simulink model "anti_windup_DC_motor_R2018a"  (R2018a)
settings: Solver=VariableStepAuto  StartTime=0.0  StopTime=200  RelTol=1e-3
libraries: simulink x1
settings Model: Creator=kjartan  LastModifiedBy=kjartan
settings DataIOCC: ReturnWorkspaceOutputs=on
settings DebuggingCC: SFMachineParentedDataDiag=error
settings SFSimCC: SimUseLocalCustomCode=on
settings RTWCC: RTWUseLocalCustomCode=on

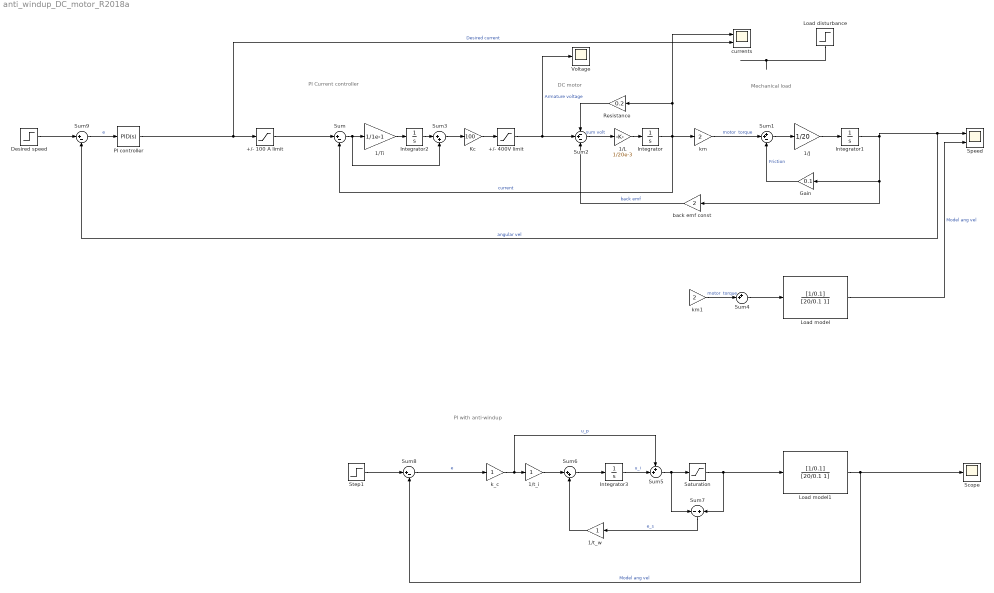
== system anti_windup_DC_motor_R2018a ==
  note: PI with anti-windup
  note: PI Current controller
  note: Mechanical load
  note: DC motor
  +/- 100 A limit : Saturate  UpperLimit=100  LowerLimit=-100
  +/- 400V limit : Saturate  UpperLimit=400  LowerLimit=-400
  1/J : Gain  Gain=1/20
  1/L : Gain  Gain=1/20e-3
  1/Ti : Gain  Gain=1/1e-1
  1/t_i : Gain
  1/t_w : Gain
  Desired speed : Step  Time=0  After=100  SampleTime=0
  Gain : Gain  Gain=0.1
  Integrator{,1..3} (4 alike) : Integrator
  Kc : Gain  Gain=100
  Load disturbance : Step  Time=10  After=10  SampleTime=0
  Load model : TransferFcn  Numerator=[1/0.1]  Denominator=[20/0.1 1]
  Load model1 : TransferFcn  Numerator=[1/0.1]  Denominator=[20/0.1 1]
  PI controller : simulink/Continuous/PID Controller  Controller=PID  Form=Ideal  TimeDomain=Continuous-time  SampleTime=-1  IntegratorMethod=Forward Euler  FilterMethod=Forward Euler  ControllerParametersSource=internal  P=10  I=1/20  D=20  UseFilter=on  N=100  TunerSelectOption=Transfer Function Based (PID Tuner App)  InitialConditionSource=internal  InitialConditionForIntegrator=0  InitialConditionForFilter=0  DifferentiatorICPrevScaledInput=0  ExternalReset=none  TrackingMode=off  Kt=1  LimitOutput=off  UpperSaturationLimit=inf  LowerSaturationLimit=-inf  LinearizeAsGain=on  AntiWindupMode=none  Kb=1  POutMin=[]  POutMax=[]  IOutMin=[]  IOutMax=[]  DOutMin=[]  DOutMax=[]  NOutMin=[]  NOutMax=[]  SumOutMin=[]  SumOutMax=[]  SaturationOutMin=[]  SaturationOutMax=[]  PParamMin=[]  PParamMax=[]  IParamMin=[]  IParamMax=[]  DParamMin=[]  DParamMax=[]  NParamMin=[]  NParamMax=[]  KbParamMin=[]  KbParamMax=[]  KtParamMin=[]  KtParamMax=[]  KbOutMin=[]  KbOutMax=[]  KtOutMin=[]  KtOutMax=[]  IntegratorOutMin=[]  IntegratorOutMax=[]  FilterOutMin=[]  FilterOutMax=[]  SumI1OutMin=[]  SumI1OutMax=[]  SumI2OutMin=[]  SumI2OutMax=[]  SumI3OutMin=[]  SumI3OutMax=[]  SumDOutMin=[]  SumDOutMax=[]  DifferentiatorOutMin=[]  DifferentiatorOutMax=[]  FilterDiffOutCoefMin=[]  FilterDiffOutCoefMax=[]  ReciprocalOutMin=[]  ReciprocalOutMax=[]  SumDenOutMin=[]  SumDenOutMax=[]  SumNumOutMin=[]  SumNumOutMax=[]  DivideOutMin=[]  DivideOutMax=[]  IntegratorContinuousStateAttributes=''  IntegratorStateMustResolveToSignalObject=off  IntegratorRTWStateStorageClass=Auto  FilterContinuousStateAttributes=''  FilterStateMustResolveToSignalObject=off  FilterRTWStateStorageClass=Auto
  Resistance : Gain  Gain=0.2
  Saturation : Saturate
  Scope : Scope
  Speed : Scope  NumInputPorts=2
  Step1 : Step  After=100  SampleTime=0
  Sum : Sum  Inputs=|+-
  Sum1 : Sum  Inputs=++-
  Sum2 : Sum  Inputs=-+-
  Sum3 : Sum  Inputs=|++
  Sum4 : Sum  Inputs=++|
  Sum5 : Sum  Inputs=++|
  Sum6 : Sum  Inputs=|++
  Sum7 : Sum  Inputs=-|+
  Sum8 : Sum  Inputs=|+-
  Sum9 : Sum  Inputs=|+-
  Voltage : Scope
  back emf const : Gain  Gain=2
  currents : Scope  NumInputPorts=2
  k_c : Gain
  km : Gain  Gain=2
  km1 : Gain  Gain=2
  wires:
  Integrator1/1 -> back emf const/1, Gain/1, Sum9/2, Speed/1  "angular vel"
  1/L/1 -> Integrator/1
  Integrator/1 -> Sum/2, currents/1, Resistance/1, km/1  "current"
  km/1 -> Sum1/2  "motor  torque"
  Sum1/1 -> 1/J/1
  1/J/1 -> Integrator1/1
  Gain/1 -> Sum1/3  "Friction"
  Sum2/1 -> 1/L/1  "sum volt"
  back emf const/1 -> Sum2/3  "back emf"
  +/- 400V limit/1 -> Voltage/1, Sum2/2  "Armature voltage"
  Resistance/1 -> Sum2/1
  Kc/1 -> +/- 400V limit/1
  Sum3/1 -> Kc/1
  Integrator2/1 -> Sum3/1
  1/Ti/1 -> Integrator2/1
  Sum/1 -> Sum3/2, 1/Ti/1
  +/- 100 A limit/1 -> Sum/1
  PI controller/1 -> currents/2, +/- 100 A limit/1  "Desired current"
  Load disturbance/1 -> ?
  Sum4/1 -> Load model/1
  Load model/1 -> Speed/2  "Model ang vel"
  Sum5/1 -> Sum7/1, Saturation/1
  Saturation/1 -> Sum7/2, Load model1/1
  Integrator3/1 -> Sum5/2  "u_i"
  Sum6/1 -> Integrator3/1
  1/t_w/1 -> Sum6/2
  Sum7/1 -> 1/t_w/1  "e_s"
  Sum8/1 -> k_c/1  "e"
  Load model1/1 -> Scope/1, Sum8/2  "Model ang vel"
  1/t_i/1 -> Sum6/1
  k_c/1 -> Sum5/1, 1/t_i/1  "u_p"
  Step1/1 -> Sum8/1
  km1/1 -> Sum4/2  "motor  torque"
  Sum9/1 -> PI controller/1  "e"
  Desired speed/1 -> Sum9/1
